simulink model "disturbances_SS_Error"  (R2021a)
settings: Solver=VariableStepAuto  StartTime=0.0  StopTime=10  RelTol=1e-3
values from neighbouring files (symbols this model uses):
  D_1 = 0    [steady_state_errors.m]
  D_2 = 0    [steady_state_errors.m]
  D_3 = 0    [steady_state_errors.m]
  D_m = 1    [steady_state_errors.m]
  d_time = 5    [steady_state_errors.m]
  K_P = 5    [disturbances_exercise_1.m]    (also in disturbances_exercise_2.m = 45; prefilters.m = 13.1; steady_state_errors.m = db2mag(-15.7))
  R = 1    [steady_state_errors.m]
undefined symbols (not defined in the file or in its folder): d_1, d_2, d_3, n_1, n_2, n_3
settings Model: Creator=dimpa  LastModifiedBy=dimpa

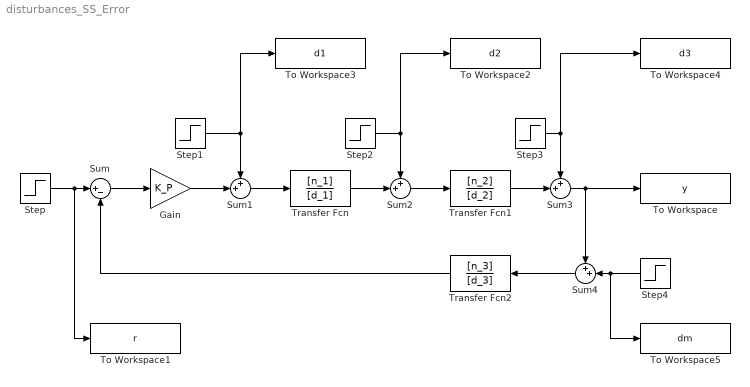
== system disturbances_SS_Error ==
  Gain : Gain  Gain=K_P
  Step : Step  Time=0  After=R  SampleTime=0
  Step1 : Step  Time=d_time  After=D_1  SampleTime=0
  Step2 : Step  Time=d_time  After=D_2  SampleTime=0
  Step3 : Step  Time=d_time  After=D_3  SampleTime=0
  Step4 : Step  Time=d_time  After=D_m  SampleTime=0
  Sum : Sum  Inputs=|+-
  Sum{1..4} (4 alike) : Sum  Inputs=++|
  To Workspace : ToWorkspace  VariableName=y  SaveFormat=Timeseries  SampleTime=-1
  To Workspace1 : ToWorkspace  VariableName=r  SaveFormat=Timeseries  SampleTime=-1
  To Workspace2 : ToWorkspace  VariableName=d2  SaveFormat=Timeseries  SampleTime=-1
  To Workspace3 : ToWorkspace  VariableName=d1  SaveFormat=Timeseries  SampleTime=-1
  To Workspace4 : ToWorkspace  VariableName=d3  SaveFormat=Timeseries  SampleTime=-1
  To Workspace5 : ToWorkspace  VariableName=dm  SaveFormat=Timeseries  SampleTime=-1
  Transfer Fcn : TransferFcn  Numerator=[n_1]  Denominator=[d_1]
  Transfer Fcn1 : TransferFcn  Numerator=[n_2]  Denominator=[d_2]
  Transfer Fcn2 : TransferFcn  Numerator=[n_3]  Denominator=[d_3]
  wires:
  Sum/1 -> Gain/1
  Gain/1 -> Sum1/2
  Sum1/1 -> Transfer Fcn/1
  Transfer Fcn/1 -> Sum2/2
  Sum2/1 -> Transfer Fcn1/1
  Transfer Fcn1/1 -> Sum3/2
  Sum3/1 -> Sum4/1, To Workspace/1
  Sum4/1 -> Transfer Fcn2/1
  Step/1 -> To Workspace1/1, Sum/1
  Transfer Fcn2/1 -> Sum/2
  Step1/1 -> To Workspace3/1, Sum1/1
  Step2/1 -> To Workspace2/1, Sum2/1
  Step3/1 -> Sum3/1, To Workspace4/1
  Step4/1 -> To Workspace5/1, Sum4/2
